simulink model "SimLab3_2_discretization"  (R2015b)
settings: Solver=ode45  SolverMode=SingleTasking  StartTime=0.0  StopTime=time  RelTol=1e-3
values from neighbouring files (symbols this model uses):
  Amplitude = 20    [Simulations_1.m]    (also in Simulations_2.m = 200; Simulations_2_disc.m; Simulations_3.m = 200; Simulations_4.m)
  Freq = 10    [Simulations_1.m]    (also in Simulations_2.m; Simulations_2_disc.m; Simulations_3.m; Simulations_4.m)
  L1 = 11.4E-3    (= 0.0114)    [Simulations_1.m]    (also in Simulations_2.m; Simulations_2_disc.m; Simulations_3.m; Simulations_4.m)
undefined symbols (not defined in the file or in its folder): dm, FB_den, FB_num, Jeq, Kemf, Km, n, R, Speed_ref_step, Ts
libraries: simulink x1
settings Model: Creator=sofianh  LastModifiedBy=es2lab2
settings DataIOCC: SaveFormat=Array
settings OptimizationCC: BlockReduction=off  BooleanDataType=off
settings DebuggingCC: SaveWithParameterizedLinksMsg=none  UnderspecifiedInitializationDetection=Classic  MergeDetectMultiDrivingBlocksExec=none  SignalResolutionControl=TryResolveAllWithWarning
settings HardwareCC: ProdBitPerPointer=32  ProdLargestAtomicFloat=None  ProdIntDivRoundTo=Undefined  ProdEndianess=Unspecified  ProdWordSize=32  ProdHWDeviceType=32-bit Generic  TargetUnknown=on
settings GRTTargetCC: GeneratePreprocessorConditionals=Disable all
settings ConfigComp: CovModelRefEnable=Off  CovSFcnEnable=off

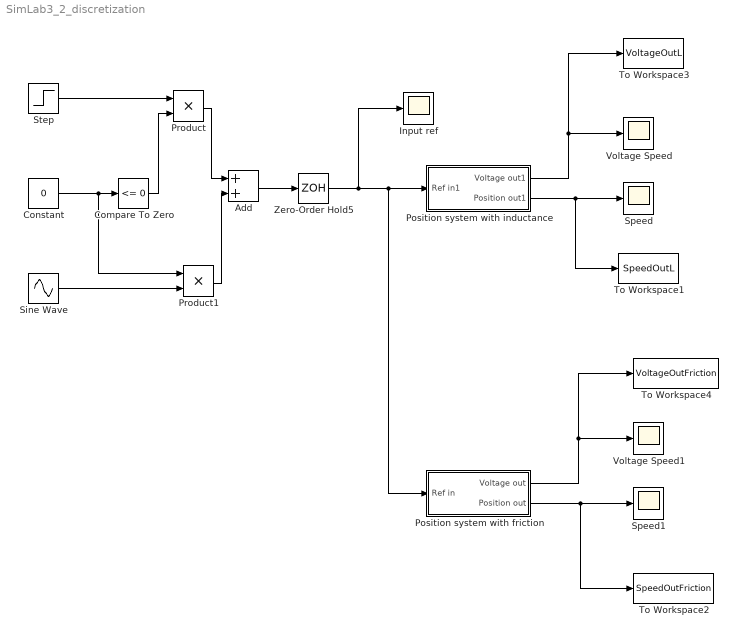
== system SimLab3_2_discretization ==
  Add : Sum
  Compare To Zero : simulink/Logic and Bit Operations/Compare To Zero  relop=<=  OutDataTypeStr=boolean
  Constant : Constant  Value=0
  Input ref : Scope
  Position system with friction : Subsystem
  Position system with inductance : Subsystem
  Product : Product
  Product1 : Product
  Sine Wave : Sin  Amplitude=Amplitude  Frequency=Freq  SampleTime=0
  Speed : Scope
  Speed1 : Scope
  Step : Step  Time=0  After=Speed_ref_step  SampleTime=0
  To Workspace1 : ToWorkspace  VariableName=SpeedOutL  SaveFormat=Structure With Time  SampleTime=Ts
  To Workspace2 : ToWorkspace  VariableName=SpeedOutFriction  SaveFormat=Structure With Time  SampleTime=Ts
  To Workspace3 : ToWorkspace  VariableName=VoltageOutL  SaveFormat=Structure With Time  SampleTime=Ts
  To Workspace4 : ToWorkspace  VariableName=VoltageOutFriction  SaveFormat=Structure With Time  SampleTime=Ts
  Voltage Speed : Scope
  Voltage Speed1 : Scope
  Zero-Order Hold5 : ZeroOrderHold  SampleTime=Ts
  wires:
  Position system with inductance/1(Voltage out1) -> To Workspace3/1, Voltage Speed/1
  Position system with inductance/2(Position out1) -> To Workspace1/1, Speed/1
  Add/1 -> Zero-Order Hold5/1
  Step/1 -> Product/1
  Constant/1 -> Product1/1, Compare To Zero/1
  Sine Wave/1 -> Product1/2
  Product/1 -> Add/1
  Product1/1 -> Add/2
  Compare To Zero/1 -> Product/2
  Position system with friction/1(Voltage out) -> To Workspace4/1, Voltage Speed1/1
  Position system with friction/2(Position out) -> To Workspace2/1, Speed1/1
  Zero-Order Hold5/1 -> Position system with inductance/1(Ref in1), Position system with friction/1(Ref in), Input ref/1

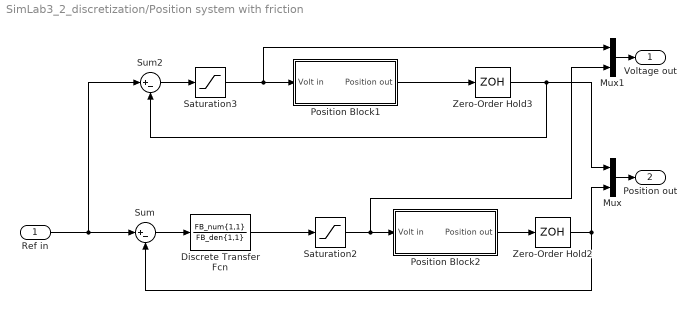
== system SimLab3_2_discretization/Position system with friction ==
  Ref in : Inport
  Discrete Transfer Fcn : DiscreteTransferFcn  Numerator=FB_num{1,1}  Denominator=FB_den{1,1}
  Mux : Mux  Inputs=2
  Mux1 : Mux  Inputs=2
  Position Block1 : Subsystem
  Position Block2 : Subsystem
  Saturation2 : Saturate  UpperLimit=24  LowerLimit=-24
  Saturation3 : Saturate  UpperLimit=24  LowerLimit=-24
  Sum : Sum  Inputs=|+-
  Sum2 : Sum  Inputs=|+-
  Zero-Order Hold2 : ZeroOrderHold  SampleTime=Ts
  Zero-Order Hold3 : ZeroOrderHold  SampleTime=Ts
  Voltage out : Outport
  Position out : Outport  Port=2
  wires:
  Sum2/1 -> Saturation3/1
  Mux/1 -> Position out/1
  Mux1/1 -> Voltage out/1
  Saturation2/1 -> Position Block2/1(Volt in), Mux1/2
  Saturation3/1 -> Position Block1/1(Volt in), Mux1/1
  Ref in/1 -> Sum/1, Sum2/1
  Zero-Order Hold3/1 -> Sum2/2, Mux/1
  Discrete Transfer Fcn/1 -> Saturation2/1
  Sum/1 -> Discrete Transfer Fcn/1
  Position Block2/1(Position out) -> Zero-Order Hold2/1
  Zero-Order Hold2/1 -> Mux/2, Sum/2
  Position Block1/1(Position out) -> Zero-Order Hold3/1

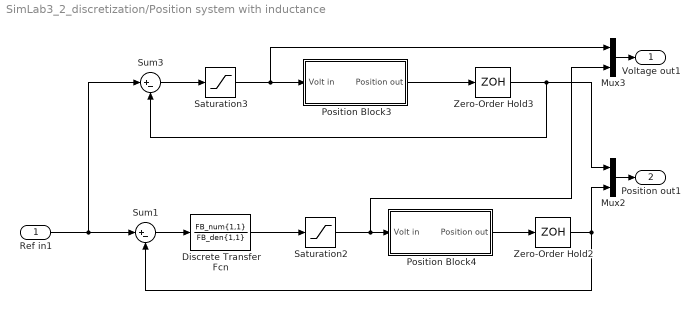
== system SimLab3_2_discretization/Position system with inductance ==
  Ref in1 : Inport
  Discrete Transfer Fcn : DiscreteTransferFcn  Numerator=FB_num{1,1}  Denominator=FB_den{1,1}
  Mux2 : Mux  Inputs=2
  Mux3 : Mux  Inputs=2
  Position Block3 : Subsystem
  Position Block4 : Subsystem
  Saturation2 : Saturate  UpperLimit=24  LowerLimit=-24
  Saturation3 : Saturate  UpperLimit=24  LowerLimit=-24
  Sum1 : Sum  Inputs=|+-
  Sum3 : Sum  Inputs=|+-
  Zero-Order Hold2 : ZeroOrderHold  SampleTime=Ts
  Zero-Order Hold3 : ZeroOrderHold  SampleTime=Ts
  Voltage out1 : Outport
  Position out1 : Outport  Port=2
  wires:
  Sum3/1 -> Saturation3/1
  Mux2/1 -> Position out1/1
  Mux3/1 -> Voltage out1/1
  Saturation2/1 -> Position Block4/1(Volt in), Mux3/2
  Saturation3/1 -> Position Block3/1(Volt in), Mux3/1
  Ref in1/1 -> Sum1/1, Sum3/1
  Zero-Order Hold3/1 -> Sum3/2, Mux2/1
  Discrete Transfer Fcn/1 -> Saturation2/1
  Sum1/1 -> Discrete Transfer Fcn/1
  Position Block4/1(Position out) -> Zero-Order Hold2/1
  Zero-Order Hold2/1 -> Mux2/2, Sum1/2
  Position Block3/1(Position out) -> Zero-Order Hold3/1

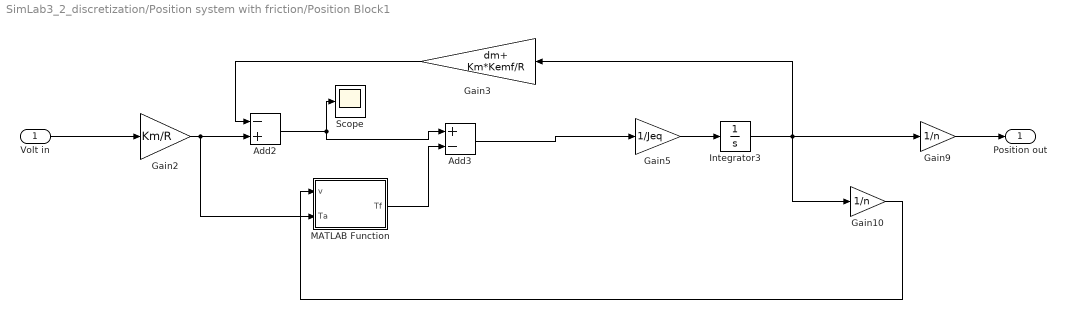
== system SimLab3_2_discretization/Position system with friction/Position Block1 ==
  Volt in : Inport
  Add2 : Sum  Inputs=-+
  Add3 : Sum  Inputs=+-
  Gain10 : Gain  Gain=1/n
  Gain2 : Gain  Gain=Km/R
  Gain3 : Gain  Gain=dm+ Km*Kemf/R
  Gain5 : Gain  Gain=1/Jeq
  Gain9 : Gain  Gain=1/n
  Integrator3 : Integrator
  MATLAB Function : MATLAB Function  TreatAsAtomicUnit=on
  Scope : Scope
  Position out : Outport
  wires:
  Gain2/1 -> MATLAB Function/2(Ta), Add2/2
  Gain3/1 -> Add2/1
  Gain5/1 -> Integrator3/1
  Gain10/1 -> MATLAB Function/1(v)
  Volt in/1 -> Gain2/1
  Add3/1 -> Gain5/1
  Add2/1 -> Add3/1, Scope/1
  MATLAB Function/1(Tf) -> Add3/2
  Integrator3/1 -> Gain9/1, Gain3/1, Gain10/1
  Gain9/1 -> Position out/1

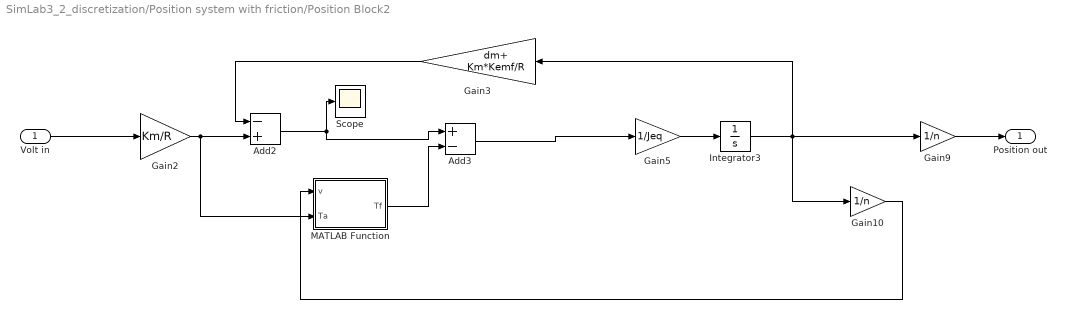
== system SimLab3_2_discretization/Position system with friction/Position Block2 ==
  Volt in : Inport
  Add2 : Sum  Inputs=-+
  Add3 : Sum  Inputs=+-
  Gain10 : Gain  Gain=1/n
  Gain2 : Gain  Gain=Km/R
  Gain3 : Gain  Gain=dm+ Km*Kemf/R
  Gain5 : Gain  Gain=1/Jeq
  Gain9 : Gain  Gain=1/n
  Integrator3 : Integrator
  MATLAB Function : MATLAB Function  TreatAsAtomicUnit=on
  Scope : Scope
  Position out : Outport
  wires:
  Gain2/1 -> MATLAB Function/2(Ta), Add2/2
  Gain3/1 -> Add2/1
  Gain5/1 -> Integrator3/1
  Gain10/1 -> MATLAB Function/1(v)
  Volt in/1 -> Gain2/1
  Add3/1 -> Gain5/1
  Add2/1 -> Add3/1, Scope/1
  MATLAB Function/1(Tf) -> Add3/2
  Integrator3/1 -> Gain9/1, Gain3/1, Gain10/1
  Gain9/1 -> Position out/1

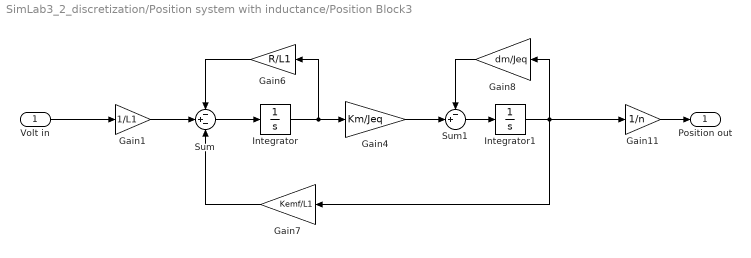
== system SimLab3_2_discretization/Position system with inductance/Position Block3 ==
  Volt in : Inport
  Gain1 : Gain  Gain=1/L1
  Gain11 : Gain  Gain=1/n
  Gain4 : Gain  Gain=Km/Jeq
  Gain6 : Gain  Gain=R/L1
  Gain7 : Gain  Gain=Kemf/L1
  Gain8 : Gain  Gain=dm/Jeq
  Integrator : Integrator
  Integrator1 : Integrator
  Sum : Sum  Inputs=-+-
  Sum1 : Sum  Inputs=-+|
  Position out : Outport
  wires:
  Gain1/1 -> Sum/2
  Sum/1 -> Integrator/1
  Integrator/1 -> Gain6/1, Gain4/1
  Sum1/1 -> Integrator1/1
  Gain4/1 -> Sum1/2
  Gain6/1 -> Sum/1
  Gain7/1 -> Sum/3
  Gain8/1 -> Sum1/1
  Gain11/1 -> Position out/1
  Volt in/1 -> Gain1/1
  Integrator1/1 -> Gain11/1, Gain8/1, Gain7/1

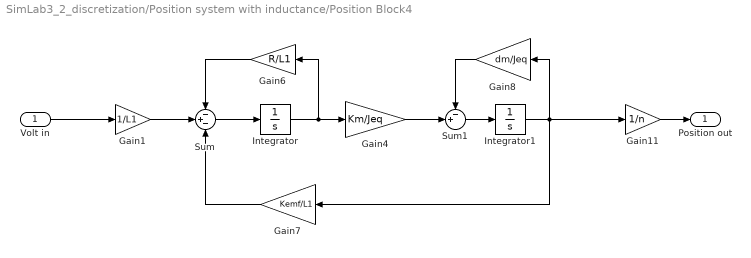
== system SimLab3_2_discretization/Position system with inductance/Position Block4 ==
  Volt in : Inport
  Gain1 : Gain  Gain=1/L1
  Gain11 : Gain  Gain=1/n
  Gain4 : Gain  Gain=Km/Jeq
  Gain6 : Gain  Gain=R/L1
  Gain7 : Gain  Gain=Kemf/L1
  Gain8 : Gain  Gain=dm/Jeq
  Integrator : Integrator
  Integrator1 : Integrator
  Sum : Sum  Inputs=-+-
  Sum1 : Sum  Inputs=-+|
  Position out : Outport
  wires:
  Gain1/1 -> Sum/2
  Sum/1 -> Integrator/1
  Integrator/1 -> Gain6/1, Gain4/1
  Sum1/1 -> Integrator1/1
  Gain4/1 -> Sum1/2
  Gain6/1 -> Sum/1
  Gain7/1 -> Sum/3
  Gain8/1 -> Sum1/1
  Gain11/1 -> Position out/1
  Volt in/1 -> Gain1/1
  Integrator1/1 -> Gain11/1, Gain8/1, Gain7/1

== matlab function SimLab3_2_discretization/Position system with friction/Position Block1/MATLAB Function ==
  data: v input; Tf output; Ta input
function Tf = fcn(v,Ta)
Tc = 1e-3;
dv = 1e-1;
if abs(v) < dv
    if abs(Ta) > Tc
        Tf = Tc*sign(Ta);
    else
        Tf = Ta;
    end
else
    Tf = Tc*sign(v);
end

== matlab function SimLab3_2_discretization/Position system with friction/Position Block2/MATLAB Function ==
  data: v input; Tf output; Ta input
function Tf = fcn(v,Ta)
Tc = 1e-3;
dv = 1e-1;
if abs(v) < dv
    if abs(Ta) > Tc
        Tf = Tc*sign(Ta);
    else
        Tf = Ta;
    end
else
    Tf = Tc*sign(v);
end
